simulink model "hw_robot_trj_ctrl_pid"  (R2020b)
settings: Solver=ode1  StartTime=0.0  StopTime=60  FixedStep=0.01  RelTol=1e-3  EnableMultiTasking=on
undefined symbols (not defined in the file): a, b, Kd, Ki, Kp
libraries: arduinolib x4, dspsigops x1
settings Model: SILPILModeSetting=veronly  ExtModeTrigDuration=2  Creator=ONLY-GOD  LastModifiedBy=ONLY-GOD
settings OptimizationCC: EnhancedBackFolding=on  PassReuseOutputArgsAs=Individual arguments  ZeroExternalMemoryAtStartup=off  ZeroInternalMemoryAtStartup=off  MaxStackSize=64  OptimizeBlockOrder=speed  DifferentSizesBufferReuse=on  OptimizationCustomize=off  EfficientTunableParamExpr=on
settings DebuggingCC: ParameterTunabilityLossMsg=error
settings HardwareCC: ProdBitPerPointer=32  ProdBitPerSizeT=32  ProdBitPerPtrDiffT=32  ProdLargestAtomicInteger=Long  ProdLargestAtomicFloat=Double  ProdWordSize=32  ProdHWDeviceType=ARM Compatible->ARM Cortex
settings SFSimCC: MATLABDynamicMemAlloc=off
settings RTWCC: Description=Embedded Coder  SystemTargetFile=ert.tlc  HardwareBoard=Arduino Due  TemplateMakefile=ert_default_tmf  Toolchain=Arduino ARM  BuildConfiguration=Faster Runs
settings CodeAppCC: ForceParamTrailComments=on  IgnoreCustomStorageClasses=off  OperatorAnnotations=on  SimulinkDataObjDesc=on  SFDataObjDesc=on  InsertBlockDesc=on
settings ERTTargetCC: SupportContinuousTime=on  SupportVariableSizeSignals=on  ExtModeTransport=3  ExtModeStaticAllocSize=24576  ExtModeMexFile=ext_xcp  ExtModeIntrfLevel=Level2 - Open

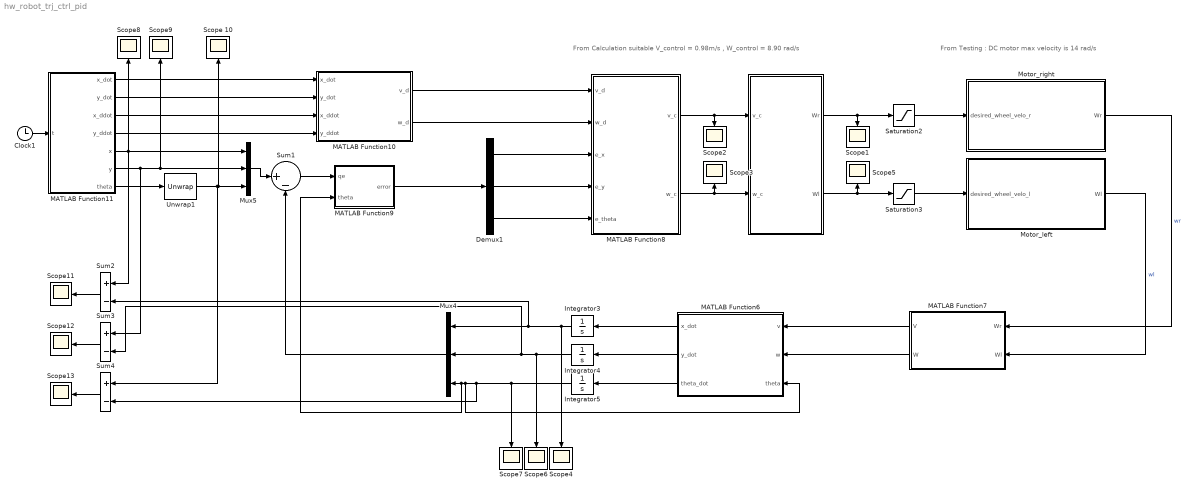
== system hw_robot_trj_ctrl_pid ==
  note: From Calculation suitable V_control = 0.98m/s , W_control = 8.90 rad/s
  note: From Testing : DC motor max velocity is 14 rad/s
  " " : MATLAB Function  TreatAsAtomicUnit=on
  Clock1 : Clock
  Demux1 : Demux  Outputs=3
  Integrator3 : Integrator
  Integrator4 : Integrator
  Integrator5 : Integrator
  MATLAB Function10 : MATLAB Function  TreatAsAtomicUnit=on
  MATLAB Function11 : MATLAB Function  TreatAsAtomicUnit=on
  MATLAB Function6 : MATLAB Function  TreatAsAtomicUnit=on
  MATLAB Function7 : MATLAB Function  TreatAsAtomicUnit=on
  MATLAB Function8 : MATLAB Function  TreatAsAtomicUnit=on
  MATLAB Function9 : MATLAB Function  TreatAsAtomicUnit=on
  Motor_left : Subsystem
  Motor_right : Subsystem
  Mux4 : Mux  Inputs=3
  Mux5 : Mux  Inputs=3
  Saturation2 : Saturate  UpperLimit=14  LowerLimit=-14
  Saturation3 : Saturate  UpperLimit=14  LowerLimit=-14
  Scope 10 : Scope
  Scope{1..9,11..13} (12 alike) : Scope
  Sum1 : Sum  Inputs=|+-
  Sum2 : Sum  Inputs=+-
  Sum3 : Sum  Inputs=+-
  Sum4 : Sum  Inputs=+-
  Unwrap1 : dspsigops/Unwrap  tol=pi  InputProcessing=Columns as channels (frame based)  running=off
  wires:
  Saturation2/1 -> Motor_right/1(desired_wheel_velo_r)
  MATLAB Function11/6(y) -> Mux5/2, Scope9/1, Sum3/1
  Unwrap1/1 -> Scope 10/1, Mux5/3, Sum4/1
  " "/2(Wl) -> Scope5/1, Saturation3/1
  Motor_right/1(Wr) -> MATLAB Function7/1(Wr)  "wr"
  Saturation3/1 -> Motor_left/1(desired_wheel_velo_l)
  Sum3/1 -> Scope12/1
  MATLAB Function10/1(v_d) -> MATLAB Function8/1(v_d)
  MATLAB Function11/5(x) -> Mux5/1, Scope8/1, Sum2/1
  MATLAB Function11/2(y_dot) -> MATLAB Function10/2(y_dot)
  Sum1/1 -> MATLAB Function9/1(qe)
  Integrator4/1 -> Sum3/2, Mux4/2, Scope6/1
  MATLAB Function11/4(y_ddot) -> MATLAB Function10/4(y_ddot)
  MATLAB Function7/2(W) -> MATLAB Function6/2(w)
  MATLAB Function7/1(V) -> MATLAB Function6/1(v)
  Mux4/1 -> Sum1/2
  Clock1/1 -> MATLAB Function11/1(t)
  MATLAB Function10/2(w_d) -> MATLAB Function8/2(w_d)
  " "/1(Wr) -> Scope1/1, Saturation2/1
  MATLAB Function11/3(x_ddot) -> MATLAB Function10/3(x_ddot)
  Sum4/1 -> Scope13/1
  MATLAB Function11/1(x_dot) -> MATLAB Function10/1(x_dot)
  MATLAB Function11/7(theta) -> Unwrap1/1
  Integrator3/1 -> Sum2/2, Mux4/1, Scope4/1
  Sum2/1 -> Scope11/1
  Motor_left/1(Wl) -> MATLAB Function7/2(Wl)  "wl"
  Mux5/1 -> Sum1/1
  MATLAB Function6/2(y_dot) -> Integrator4/1
  MATLAB Function8/2(w_c) -> Scope3/1, " "/2(w_c)
  Demux1/3 -> MATLAB Function8/5(e_theta)
  MATLAB Function6/1(x_dot) -> Integrator3/1
  Integrator5/1 -> Sum4/2, Mux4/3, MATLAB Function9/2(theta), MATLAB Function6/3(theta), Scope7/1
  MATLAB Function9/1(error) -> Demux1/1
  MATLAB Function6/3(theta_dot) -> Integrator5/1
  MATLAB Function8/1(v_c) -> Scope2/1, " "/1(v_c)
  Demux1/2 -> MATLAB Function8/4(e_y)
  Demux1/1 -> MATLAB Function8/3(e_x)

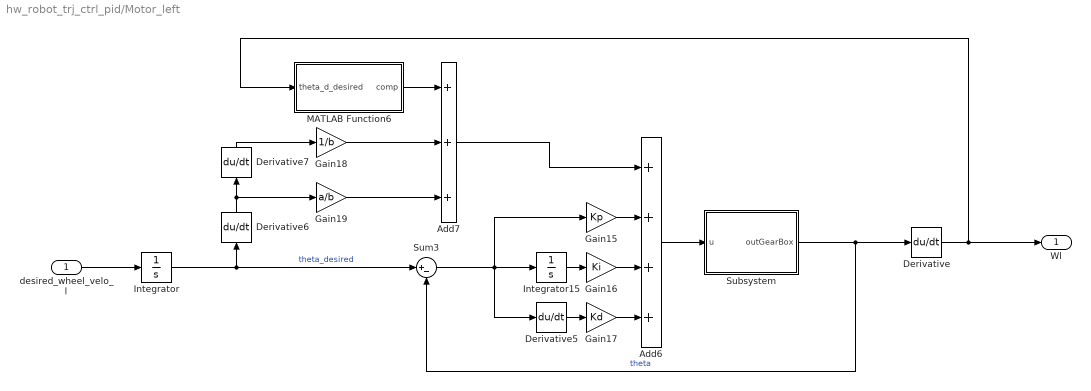
== system hw_robot_trj_ctrl_pid/Motor_left ==
  desired_wheel_velo_l : Inport
  Add6 : Sum  Inputs=++++
  Add7 : Sum  Inputs=+++
  Derivative{,5..7} (4 alike) : Derivative
  Gain15 : Gain  Gain=Kp
  Gain16 : Gain  Gain=Ki
  Gain17 : Gain  Gain=Kd
  Gain18 : Gain  Gain=1/b
  Gain19 : Gain  Gain=a/b
  Integrator : Integrator
  Integrator15 : Integrator
  MATLAB Function6 : MATLAB Function  TreatAsAtomicUnit=on
  Subsystem : Subsystem
  Sum3 : Sum  Inputs=|+-
  Wl : Outport
  wires:
  Sum3/1 -> Derivative5/1, Integrator15/1, Gain15/1
  Integrator/1 -> Derivative6/1, Sum3/1  "theta_desired"
  Derivative5/1 -> Gain17/1
  Gain19/1 -> Add7/3
  Gain15/1 -> Add6/2
  MATLAB Function6/1(comp) -> Add7/1
  Add7/1 -> Add6/1
  Derivative7/1 -> Gain18/1
  Integrator15/1 -> Gain16/1
  Gain16/1 -> Add6/3
  Subsystem/1(outGearBox) -> Derivative/1, Sum3/2  "theta"
  Gain18/1 -> Add7/2
  Derivative6/1 -> Derivative7/1, Gain19/1
  Gain17/1 -> Add6/4
  desired_wheel_velo_l/1 -> Integrator/1
  Add6/1 -> Subsystem/1(u)
  Derivative/1 -> MATLAB Function6/1(theta_d_desired), Wl/1

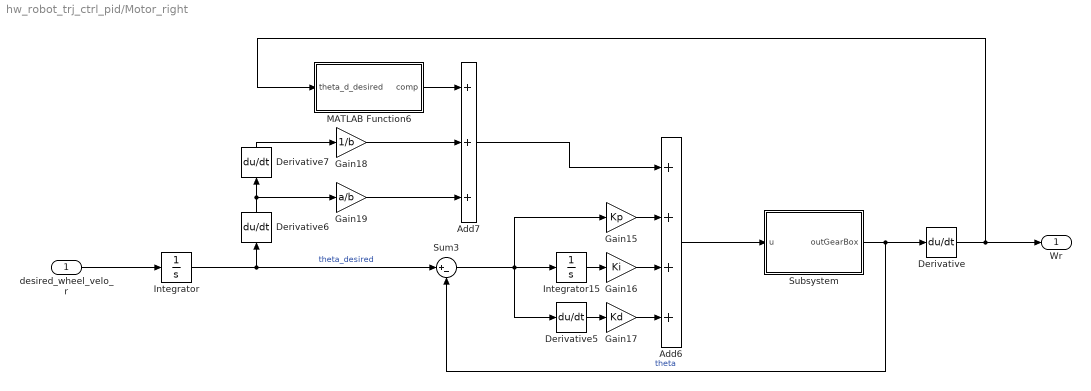
== system hw_robot_trj_ctrl_pid/Motor_right ==
  desired_wheel_velo_r : Inport
  Add6 : Sum  Inputs=++++
  Add7 : Sum  Inputs=+++
  Derivative{,5..7} (4 alike) : Derivative
  Gain15 : Gain  Gain=Kp
  Gain16 : Gain  Gain=Ki
  Gain17 : Gain  Gain=Kd
  Gain18 : Gain  Gain=1/b
  Gain19 : Gain  Gain=a/b
  Integrator : Integrator
  Integrator15 : Integrator
  MATLAB Function6 : MATLAB Function  TreatAsAtomicUnit=on
  Subsystem : Subsystem
  Sum3 : Sum  Inputs=|+-
  Wr : Outport
  wires:
  desired_wheel_velo_r/1 -> Integrator/1
  Add7/1 -> Add6/1
  Gain18/1 -> Add7/2
  Subsystem/1(outGearBox) -> Derivative/1, Sum3/2  "theta"
  Gain16/1 -> Add6/3
  Gain19/1 -> Add7/3
  Integrator15/1 -> Gain16/1
  Derivative7/1 -> Gain18/1
  Gain17/1 -> Add6/4
  Gain15/1 -> Add6/2
  Derivative5/1 -> Gain17/1
  Sum3/1 -> Gain15/1, Integrator15/1, Derivative5/1
  Add6/1 -> Subsystem/1(u)
  Derivative6/1 -> Gain19/1, Derivative7/1
  Integrator/1 -> Sum3/1, Derivative6/1  "theta_desired"
  MATLAB Function6/1(comp) -> Add7/1
  Derivative/1 -> MATLAB Function6/1(theta_d_desired), Wr/1

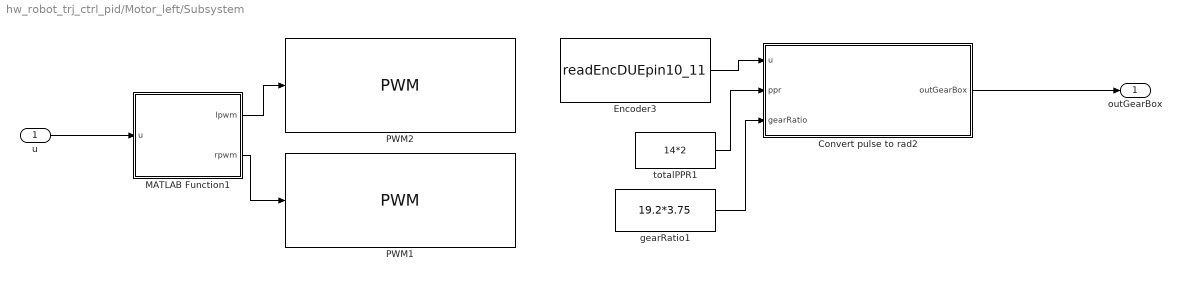
== system hw_robot_trj_ctrl_pid/Motor_left/Subsystem ==
  u : Inport
  Convert pulse to rad2 : MATLAB Function  TreatAsAtomicUnit=on
  Encoder3 : S-Function  InitFcn=try, set_param(gcb,'FunctionName','readEncDUEpin10_11'), end  FunctionName=readEncDUEpin10_11  SFunctionModules=readEncDUEpin10_11_wrapper  SFunctionDeploymentMode=off  EnableBusSupport=off  mask(S-Function Builder){}
      mask help: Simulink:masks:SFunctionBuilder_MD
      mask init:
      | val = [[.9  0.75 0.75 1 1 .9 .9 1]',[1 1 0.75 0.75 .9 .9 1 .9]'];try , sys = get_param(gcb,'SfunBuilderFcnName');if isempty(sys), sys = get_param(gcb,'FunctionName'); end,catch, sys = get_param(gcb,'FunctionName'); end
      settings: CopyFcn=set_param(gcbh,'LinkStatus','none')  PreSaveFcn=try, set_param(gcb,'FunctionName','readEncDUEpin10_11'), end  OpenFcn=sfunctionwizard(gcbh)
      mask Display: plot(val(:,1),val(:,2)),disp(sys),port_label('output',1,'countt')
  MATLAB Function1 : MATLAB Function  TreatAsAtomicUnit=on
  PWM1 : arduinolib/PWM  pinNumber=4  frequencyType=Default  desiredFrequency=490.2  achievableFrequency=490.2
  PWM2 : arduinolib/PWM  pinNumber=5  frequencyType=Default  desiredFrequency=490.2  achievableFrequency=490.2
  gearRatio1 : Constant  Value=19.2*3.75
  totalPPR1 : Constant  Value=14*2
  outGearBox : Outport
  wires:
  Encoder3/1 -> Convert pulse to rad2/1(u)
  totalPPR1/1 -> Convert pulse to rad2/2(ppr)
  gearRatio1/1 -> Convert pulse to rad2/3(gearRatio)
  Convert pulse to rad2/1(outGearBox) -> outGearBox/1
  MATLAB Function1/1(lpwm) -> PWM2/1
  MATLAB Function1/2(rpwm) -> PWM1/1
  u/1 -> MATLAB Function1/1(u)

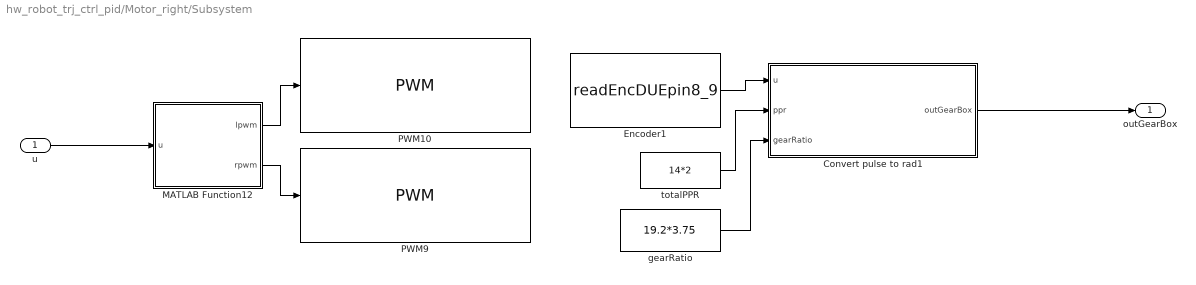
== system hw_robot_trj_ctrl_pid/Motor_right/Subsystem ==
  u : Inport
  Convert pulse to rad1 : MATLAB Function  TreatAsAtomicUnit=on
  Encoder1 : S-Function  InitFcn=try, set_param(gcb,'FunctionName','readEncDUEpin8_9'), end  FunctionName=readEncDUEpin8_9  SFunctionModules=readEncDUEpin8_9_wrapper  SFunctionDeploymentMode=off  EnableBusSupport=off  mask(S-Function Builder){}
      mask help: Simulink:masks:SFunctionBuilder_MD
      mask init: same as hw_robot_trj_ctrl_pid/Motor_left/Subsystem/Encoder3
      settings: CopyFcn=set_param(gcbh,'LinkStatus','none')  PreSaveFcn=try, set_param(gcb,'FunctionName','readEncDUEpin8_9'), end  OpenFcn=sfunctionwizard(gcbh)
      mask Display: plot(val(:,1),val(:,2)),disp(sys),port_label('output',1,'count')
  MATLAB Function12 : MATLAB Function  TreatAsAtomicUnit=on
  PWM10 : arduinolib/PWM  pinNumber=7  frequencyType=Default  desiredFrequency=490.2  achievableFrequency=490.2
  PWM9 : arduinolib/PWM  pinNumber=6  frequencyType=Default  desiredFrequency=490.2  achievableFrequency=490.2
  gearRatio : Constant  Value=19.2*3.75
  totalPPR : Constant  Value=14*2
  outGearBox : Outport
  wires:
  gearRatio/1 -> Convert pulse to rad1/3(gearRatio)
  MATLAB Function12/2(rpwm) -> PWM9/1
  MATLAB Function12/1(lpwm) -> PWM10/1
  totalPPR/1 -> Convert pulse to rad1/2(ppr)
  Encoder1/1 -> Convert pulse to rad1/1(u)
  Convert pulse to rad1/1(outGearBox) -> outGearBox/1
  u/1 -> MATLAB Function12/1(u)

== matlab function hw_robot_trj_ctrl_pid/Motor_right/Subsystem/Convert pulse to rad1 ==
  settings: updateMethod=DISCRETE
  data: u input; ppr input; gearRatio input; outGearBox output
function outGearBox = fcn(u,ppr,gearRatio)

persistent counter_num over_flag
if(isempty(counter_num)), counter_num = 0;end
if(isempty(over_flag)), over_flag = 0;end
pulse2radian = 2*pi/ppr; % 1 pulse = ?? radian

if(double(u) - counter_num > 40000), over_flag = over_flag-1;
elseif(double(u) - counter_num < -40000), over_flag = over_flag+1;
end

inGearBox = (double(u)+over_flag*(2^32 -1))*pulse2radian; 
outGearBox = inGearBox/gearRatio;
counter_num = double(u) ;

== matlab function hw_robot_trj_ctrl_pid/Motor_right/Subsystem/MATLAB Function12 ==
  data: u input; lpwm output; rpwm output
function [lpwm,rpwm] = fcn(u)

Vmax = 22.9;
pwm = u*254/Vmax;
if pwm > 0
    lpwm = pwm;
    rpwm = 0;
elseif pwm < 0
    lpwm = 0;
    rpwm = abs(pwm);
else
    lpwm = 0;
    rpwm = 0;
end

== matlab function hw_robot_trj_ctrl_pid/Motor_right/MATLAB Function6 ==
  settings: updateMethod=DISCRETE
  data: theta_d_desired input; comp output
function comp = fcn(theta_d_desired)

b = 17.35; c = 5.63; %+ 0.3*rand;
comp = c/b*sign(theta_d_desired);

== matlab function hw_robot_trj_ctrl_pid/Motor_left/MATLAB Function6 ==
  settings: updateMethod=DISCRETE
  data: theta_d_desired input; comp output
function comp = fcn(theta_d_desired)

b = 17.35; c = 5.63; %+ 0.3*rand;
comp = c/b*sign(theta_d_desired);

== matlab function hw_robot_trj_ctrl_pid/  ==
  data: v_c input; Wr output; w_c input; Wl output
function [Wr, Wl] = M_inv(v_c, w_c)
r = 0.07;      %wheel radius
b = 0.22;      %length from wheel to wheel

Wr = ((2*v_c)+(w_c*b))/(2*r);
Wl = ((2*v_c)-(w_c*b))/(2*r);

== matlab function hw_robot_trj_ctrl_pid/MATLAB Function10 ==
  data: x_dot input; v_d output; w_d output; y_dot input; x_ddot input; y_ddot input
function [v_d,w_d] = fcn(x_dot,y_dot,x_ddot,y_ddot)

v_d = sqrt(x_dot^2 + y_dot^2);
w_d = ((x_dot*y_ddot)-(y_dot*x_ddot))/((x_dot^2 + y_dot^2));

== matlab function hw_robot_trj_ctrl_pid/MATLAB Function11 ==
  data: x_dot output; y_dot output; x_ddot output; y_ddot output; x output; t input; y output; theta output
function [x_dot,y_dot,x_ddot,y_ddot,x,y,theta] = ref(t)

f = 2*pi*0.01;
r = 4;

x = r*cos(f*t);
y = r*sin(f*t);

x_dot = -r*f*sin(f*t);
y_dot = r*f*cos(f*t);

theta = atan2(y_dot,x_dot);

x_ddot = -r*f^2*cos(f*t);
y_ddot = -r*f^2*sin(f*t);

== matlab function hw_robot_trj_ctrl_pid/MATLAB Function6 ==
  data: v input; x_dot output; w input; y_dot output; theta_dot output; theta input
function [x_dot,y_dot,theta_dot]= kinematic(v,w,theta)
x_dot = v*cos(theta);
y_dot = v*sin(theta);
theta_dot = w;

== matlab function hw_robot_trj_ctrl_pid/MATLAB Function7 ==
  data: Wr input; V output; Wl input; W output
function [V,W]= fcn(Wr,Wl)
r = 0.07;      %wheel radius
b = 0.22;      %length from wheel to wheel

V = r*(Wr/2) + r*(Wl/2);
W = r*(Wr/b) - r*(Wl/b);

== matlab function hw_robot_trj_ctrl_pid/MATLAB Function8 ==
  data: v_d input; v_c output; w_d input; e_x input; e_y input; e_theta input; w_c output
function [v_c,w_c] =  bckstep(v_d, w_d, e_x, e_y, e_theta)            
%Experiment 1:
% k1 = 0.1;
% k2 = 2 ;
% k3 = 1 ;

% control gain
k1 = 0.1;
k2 = 2 ;
k3 = 1 ;

v_c = k1*e_x + v_d*cos(e_theta);
w_c = w_d + k2*v_d*e_y + k3*v_d*sin(e_theta);

== matlab function hw_robot_trj_ctrl_pid/MATLAB Function9 ==
  data: qe input; error output; theta input
function error = rotation(qe,theta)

T = [cos(theta) , sin(theta) , 0 ;
    -sin(theta) , cos(theta) , 0 ;
         0      ,     0      , 1 ];
     
error = T*qe;

== matlab function hw_robot_trj_ctrl_pid/Motor_left/Subsystem/Convert pulse to rad2 ==
  settings: updateMethod=DISCRETE
  data: u input; ppr input; gearRatio input; outGearBox output
function outGearBox = fcn(u,ppr,gearRatio)

persistent counter_num over_flag
if(isempty(counter_num)), counter_num = 0;end
if(isempty(over_flag)), over_flag = 0;end
pulse2radian = 2*pi/ppr; % 1 pulse = ?? radian

if(double(u) - counter_num > 40000), over_flag = over_flag-1;
elseif(double(u) - counter_num < -40000), over_flag = over_flag+1;
end

inGearBox = (double(u)+over_flag*(2^32 -1))*pulse2radian; 
outGearBox = inGearBox/gearRatio;
counter_num = double(u) ;

== matlab function hw_robot_trj_ctrl_pid/Motor_left/Subsystem/MATLAB Function1 ==
  data: u input; lpwm output; rpwm output
function [lpwm,rpwm] = fcn(u)

Vmax = 22.9;
pwm = u*254/Vmax;
if pwm > 0
    lpwm = pwm;
    rpwm = 0;
elseif pwm < 0
    lpwm = 0;
    rpwm = abs(pwm);
else
    lpwm = 0;
    rpwm = 0;
end
